simulink model "QuadRotorController_SIL"  (R2014b)
settings: Solver=FixedStepDiscrete  StartTime=0.0  StopTime=15  FixedStep=0.01  RelTol=1e-3
libraries: simulink x6
settings Model: Creator=ppreethi  LastModifiedBy=syoon
settings DataIOCC: SaveOutput=off  SaveTime=off
settings OptimizationCC: OptimizeModelRefInitCode=on  LifeSpan=Inf
settings DebuggingCC: UnderspecifiedInitializationDetection=Classic  MergeDetectMultiDrivingBlocksExec=none  StateNameClashWarn=warning
settings RTWCC: SystemTargetFile=ert.tlc  TemplateMakefile=ert_default_tmf  Description=Embedded Coder  GenerateReport=on  ProcessScript=ert_make_rtw_hook  IncludeHyperlinkInReport=on  LaunchReport=on  PortableWordSizes=on  CreateSILPILBlock=SIL  GenerateTraceInfo=on  GenerateTraceReport=on  GenerateTraceReportSl=on  GenerateTraceReportSf=on  GenerateTraceReportEml=on  GenerateCodeMetricsReport=on
settings CodeAppCC: IgnoreCustomStorageClasses=off
settings ERTTargetCC: GenerateSampleERTMain=on  SupportAbsoluteTime=off  SupportNonFinite=off  SupportComplex=off  ERTCustomFileTemplate=example_file_process.tlc
settings SimscapeCC: SelectedTab=SimMechanics2G

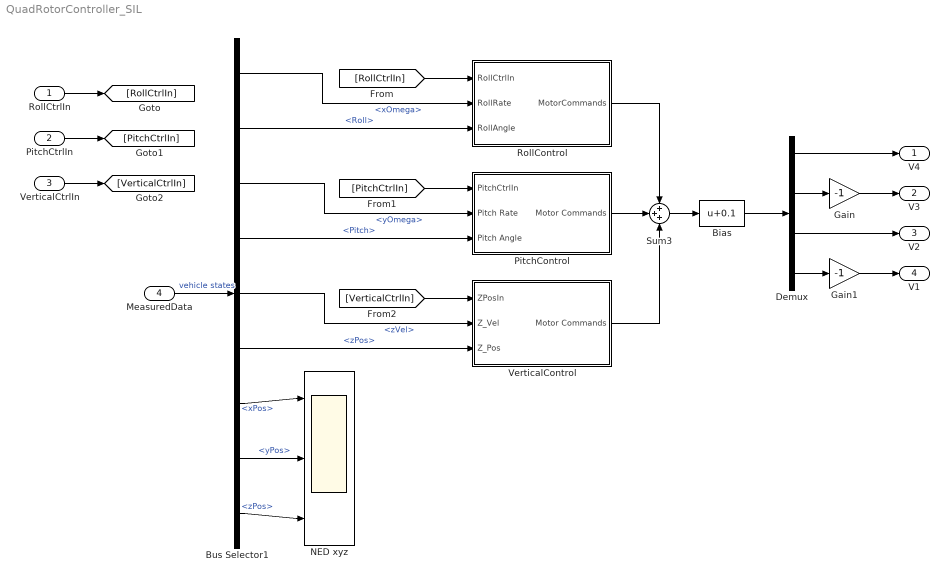
== system QuadRotorController_SIL ==
  RollCtrlIn : Inport  OutDataTypeStr=double  PortDimensions=1  SampleTime=[0.01,0]
  PitchCtrlIn : Inport  Port=2  OutDataTypeStr=double  PortDimensions=1  SampleTime=[0.01,0]
  VerticalCtrlIn : Inport  Port=3  OutDataTypeStr=double  PortDimensions=1  SampleTime=[0.01,0]
  MeasuredData : Inport  Port=4  OutDataTypeStr=Bus: VehicleStates  PortDimensions=1  SampleTime=0.01  BusOutputAsStruct=on
  Bias : Bias  Bias=0.1
  Bus Selector1 : BusSelector  OutputSignals=BodyState.AngularRate.xOmega,BodyState.Attitude.Roll,BodyState.AngularRate.yOmega,BodyState.Attitude.Pitch,BodyState.Velocity.zVel,BodyState.Position.zPos,NEDState.Position.xPos,NEDState.Position.yPos,NEDState.Position.zPos
  Demux : Demux
  Gain : Gain  Gain=-1
  Gain1 : Gain  Gain=-1
  NED xyz : Scope  NumInputPorts=3
      settings: YMin=-0.06~0.01~-1.15  YMax=0.08~0.035~-1.1  SaveName=ScopeData10
  PitchControl : Subsystem
  RollControl : Subsystem
  Sum3 : Sum  Inputs=+++
  VerticalControl : Subsystem
  V4 : Outport  OutDataTypeStr=double  PortDimensions=1  SampleTime=[0.01,0]
  V3 : Outport  Port=2  OutDataTypeStr=double  PortDimensions=1  SampleTime=[0.01,0]
  V2 : Outport  Port=3  OutDataTypeStr=double  PortDimensions=1  SampleTime=[0.01,0]
  V1 : Outport  Port=4  OutDataTypeStr=double  PortDimensions=1  SampleTime=[0.01,0]
  wires:
  Demux/3 -> V2/1
  Gain/1 -> V3/1
  Demux/2 -> Gain/1
  MeasuredData/1 -> Bus Selector1/1  "vehicle states"
  Demux/1 -> V4/1
  Gain1/1 -> V1/1
  Demux/4 -> Gain1/1
  Bus Selector1/1 -> RollControl/2(RollRate)  "<xOmega>"
  Bus Selector1/2 -> RollControl/3(RollAngle)  "<Roll>"
  Bus Selector1/3 -> PitchControl/2(Pitch Rate)  "<yOmega>"
  Bus Selector1/4 -> PitchControl/3(Pitch Angle)  "<Pitch>"
  Bus Selector1/5 -> VerticalControl/2(Z_Vel)  "<zVel>"
  Bus Selector1/6 -> VerticalControl/3(Z_Pos)  "<zPos>"
  VerticalControl/1(Motor Commands) -> Sum3/3
  Bus Selector1/8 -> NED xyz/2  "<yPos>"
  Bus Selector1/9 -> NED xyz/3  "<zPos>"
  Bus Selector1/7 -> NED xyz/1  "<xPos>"
  PitchControl/1(Motor Commands) -> Sum3/2
  RollControl/1(MotorCommands) -> Sum3/1
  Sum3/1 -> Bias/1
  Bias/1 -> Demux/1
  [VerticalCtrlIn] -> VerticalControl/1(ZPosIn)
  [RollCtrlIn] -> RollControl/1(RollCtrlIn)
  RollCtrlIn/1 -> [RollCtrlIn]
  PitchCtrlIn/1 -> [PitchCtrlIn]
  VerticalCtrlIn/1 -> [VerticalCtrlIn]
  [PitchCtrlIn] -> PitchControl/1(PitchCtrlIn)

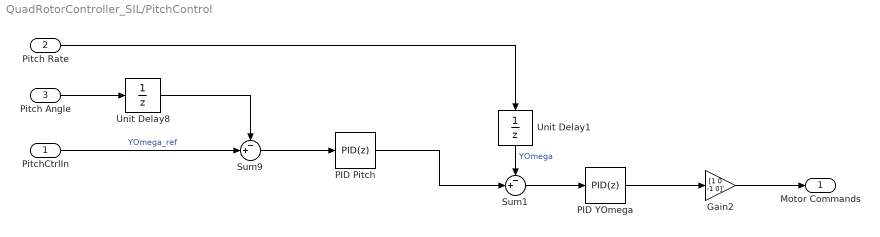
== system QuadRotorController_SIL/PitchControl ==
  PitchCtrlIn : Inport
  Pitch Rate : Inport  Port=2
  Pitch Angle : Inport  Port=3
  " PID Pitch" : simulink/Continuous/PID Controller  Controller=PID  TimeDomain=Discrete-time  SampleTime=0.01  IntegratorMethod=Forward Euler  FilterMethod=Forward Euler  Form=Parallel  P=14.2867013608458  I=2.05995750811476  D=0.849494683603069  N=180.961333470231  InitialConditionSource=internal  InitialConditionForIntegrator=0  InitialConditionForFilter=0  ExternalReset=none  LimitOutput=on  UpperSaturationLimit=10*pi/180  LowerSaturationLimit=-10*pi/180  LinearizeAsGain=on  AntiWindupMode=clamping  Kb=1  TrackingMode=off  Kt=1  PParamMin=[]  PParamMax=[]  IParamMin=[]  IParamMax=[]  DParamMin=[]  DParamMax=[]  NParamMin=[]  NParamMax=[]  KbParamMin=[]  KbParamMax=[]  KtParamMin=[]  KtParamMax=[]  POutMin=[]  POutMax=[]  IOutMin=[]  IOutMax=[]  DOutMin=[]  DOutMax=[]  NOutMin=[]  NOutMax=[]  KbOutMin=[]  KbOutMax=[]  KtOutMin=[]  KtOutMax=[]  IntegratorOutMin=[]  IntegratorOutMax=[]  FilterOutMin=[]  FilterOutMax=[]  SumOutMin=[]  SumOutMax=[]  SumI1OutMin=[]  SumI1OutMax=[]  SumI2OutMin=[]  SumI2OutMax=[]  SumI3OutMin=[]  SumI3OutMax=[]  SumDOutMin=[]  SumDOutMax=[]  SaturationOutMin=[]  SaturationOutMax=[]  IntegratorContinuousStateAttributes=''  IntegratorStateMustResolveToSignalObject=off  IntegratorRTWStateStorageClass=Auto  FilterContinuousStateAttributes=''  FilterStateMustResolveToSignalObject=off  FilterRTWStateStorageClass=Auto  DifferentiatorICPrevScaledInput=0  DifferentiatorOutMin=[]  DifferentiatorOutMax=[]  UseFilter=on
  Gain2 : Gain  Gain=[1 0 -1 0]'
  PID YOmega : simulink/Continuous/PID Controller  Controller=PID  TimeDomain=Discrete-time  SampleTime=0.01  IntegratorMethod=Forward Euler  FilterMethod=Forward Euler  Form=Parallel  P=-0.164246341346142  I=-0.0185275176619116  D=-0.032581970187069  N=81.8253210225443  InitialConditionSource=internal  InitialConditionForIntegrator=0  InitialConditionForFilter=0  ExternalReset=none  LimitOutput=on  UpperSaturationLimit=20*(pi/180)  LowerSaturationLimit=-20*(pi/180)  LinearizeAsGain=on  AntiWindupMode=clamping  Kb=1  TrackingMode=off  Kt=1  PParamMin=[]  PParamMax=[]  IParamMin=[]  IParamMax=[]  DParamMin=[]  DParamMax=[]  NParamMin=[]  NParamMax=[]  KbParamMin=[]  KbParamMax=[]  KtParamMin=[]  KtParamMax=[]  POutMin=[]  POutMax=[]  IOutMin=[]  IOutMax=[]  DOutMin=[]  DOutMax=[]  NOutMin=[]  NOutMax=[]  KbOutMin=[]  KbOutMax=[]  KtOutMin=[]  KtOutMax=[]  IntegratorOutMin=[]  IntegratorOutMax=[]  FilterOutMin=[]  FilterOutMax=[]  SumOutMin=[]  SumOutMax=[]  SumI1OutMin=[]  SumI1OutMax=[]  SumI2OutMin=[]  SumI2OutMax=[]  SumI3OutMin=[]  SumI3OutMax=[]  SumDOutMin=[]  SumDOutMax=[]  SaturationOutMin=[]  SaturationOutMax=[]  IntegratorContinuousStateAttributes=''  IntegratorStateMustResolveToSignalObject=off  IntegratorRTWStateStorageClass=Auto  FilterContinuousStateAttributes=''  FilterStateMustResolveToSignalObject=off  FilterRTWStateStorageClass=Auto  DifferentiatorICPrevScaledInput=0  DifferentiatorOutMin=[]  DifferentiatorOutMax=[]  UseFilter=on
  Sum1 : Sum  Inputs=-+|
  Sum9 : Sum  Inputs=-+|
  Unit Delay1 : UnitDelay  SampleTime=0.01
  Unit Delay8 : UnitDelay  SampleTime=0.01
  Motor Commands : Outport
  wires:
  Sum1/1 -> PID YOmega/1
  Pitch Rate/1 -> Unit Delay1/1
  Unit Delay1/1 -> Sum1/1  "YOmega"
  Pitch Angle/1 -> Unit Delay8/1
  Unit Delay8/1 -> Sum9/1
  PitchCtrlIn/1 -> Sum9/2  "YOmega_ref"
  Sum9/1 -> " PID Pitch"/1
  " PID Pitch"/1 -> Sum1/2
  PID YOmega/1 -> Gain2/1
  Gain2/1 -> Motor Commands/1

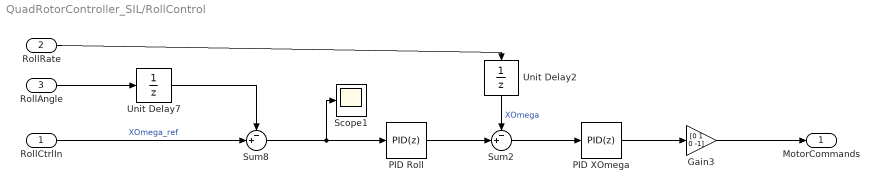
== system QuadRotorController_SIL/RollControl ==
  RollCtrlIn : Inport
  RollRate : Inport  Port=2
  RollAngle : Inport  Port=3
  " PID Roll" : simulink/Continuous/PID Controller  Controller=PID  TimeDomain=Discrete-time  SampleTime=0.01  IntegratorMethod=Forward Euler  FilterMethod=Forward Euler  Form=Parallel  P=11.7648822632631  I=1.23976611873708  D=0.415028302530751  N=77.6264609638492  InitialConditionSource=internal  InitialConditionForIntegrator=0  InitialConditionForFilter=0  ExternalReset=none  LimitOutput=on  UpperSaturationLimit=10*pi/180  LowerSaturationLimit=-10*pi/180  LinearizeAsGain=on  AntiWindupMode=clamping  Kb=1  TrackingMode=off  Kt=1  PParamMin=[]  PParamMax=[]  IParamMin=[]  IParamMax=[]  DParamMin=[]  DParamMax=[]  NParamMin=[]  NParamMax=[]  KbParamMin=[]  KbParamMax=[]  KtParamMin=[]  KtParamMax=[]  POutMin=[]  POutMax=[]  IOutMin=[]  IOutMax=[]  DOutMin=[]  DOutMax=[]  NOutMin=[]  NOutMax=[]  KbOutMin=[]  KbOutMax=[]  KtOutMin=[]  KtOutMax=[]  IntegratorOutMin=[]  IntegratorOutMax=[]  FilterOutMin=[]  FilterOutMax=[]  SumOutMin=[]  SumOutMax=[]  SumI1OutMin=[]  SumI1OutMax=[]  SumI2OutMin=[]  SumI2OutMax=[]  SumI3OutMin=[]  SumI3OutMax=[]  SumDOutMin=[]  SumDOutMax=[]  SaturationOutMin=[]  SaturationOutMax=[]  IntegratorContinuousStateAttributes=''  IntegratorStateMustResolveToSignalObject=off  IntegratorRTWStateStorageClass=Auto  FilterContinuousStateAttributes=''  FilterStateMustResolveToSignalObject=off  FilterRTWStateStorageClass=Auto  DifferentiatorICPrevScaledInput=0  DifferentiatorOutMin=[]  DifferentiatorOutMax=[]  UseFilter=on
  " PID XOmega" : simulink/Continuous/PID Controller  Controller=PID  TimeDomain=Discrete-time  SampleTime=0.01  IntegratorMethod=Forward Euler  FilterMethod=Forward Euler  Form=Parallel  P=-0.159149757061445  I=-0.0204269947322092  D=-0.0384500404495734  N=88.6017486491099  InitialConditionSource=internal  InitialConditionForIntegrator=0  InitialConditionForFilter=0  ExternalReset=none  LimitOutput=on  UpperSaturationLimit=20*(pi/180)  LowerSaturationLimit=-20*(pi/180)  LinearizeAsGain=on  AntiWindupMode=clamping  Kb=1  TrackingMode=off  Kt=1  PParamMin=[]  PParamMax=[]  IParamMin=[]  IParamMax=[]  DParamMin=[]  DParamMax=[]  NParamMin=[]  NParamMax=[]  KbParamMin=[]  KbParamMax=[]  KtParamMin=[]  KtParamMax=[]  POutMin=[]  POutMax=[]  IOutMin=[]  IOutMax=[]  DOutMin=[]  DOutMax=[]  NOutMin=[]  NOutMax=[]  KbOutMin=[]  KbOutMax=[]  KtOutMin=[]  KtOutMax=[]  IntegratorOutMin=[]  IntegratorOutMax=[]  FilterOutMin=[]  FilterOutMax=[]  SumOutMin=[]  SumOutMax=[]  SumI1OutMin=[]  SumI1OutMax=[]  SumI2OutMin=[]  SumI2OutMax=[]  SumI3OutMin=[]  SumI3OutMax=[]  SumDOutMin=[]  SumDOutMax=[]  SaturationOutMin=[]  SaturationOutMax=[]  IntegratorContinuousStateAttributes=''  IntegratorStateMustResolveToSignalObject=off  IntegratorRTWStateStorageClass=Auto  FilterContinuousStateAttributes=''  FilterStateMustResolveToSignalObject=off  FilterRTWStateStorageClass=Auto  DifferentiatorICPrevScaledInput=0  DifferentiatorOutMin=[]  DifferentiatorOutMax=[]  UseFilter=on
  Gain3 : Gain  Gain=[0 1 0 -1]
  Scope1 : Scope
      settings: YMin=-3.5  YMax=3.5  SaveName=ScopeData5
  Sum2 : Sum  Inputs=-+|
  Sum8 : Sum  Inputs=-+|
  Unit Delay2 : UnitDelay  SampleTime=0.01
  Unit Delay7 : UnitDelay  SampleTime=0.01
  MotorCommands : Outport
  wires:
  Gain3/1 -> MotorCommands/1
  Unit Delay2/1 -> Sum2/1  "XOmega"
  RollRate/1 -> Unit Delay2/1
  Sum2/1 -> " PID XOmega"/1
  " PID XOmega"/1 -> Gain3/1
  " PID Roll"/1 -> Sum2/2
  Unit Delay7/1 -> Sum8/1
  Sum8/1 -> " PID Roll"/1, Scope1/1
  RollAngle/1 -> Unit Delay7/1
  RollCtrlIn/1 -> Sum8/2  "XOmega_ref"

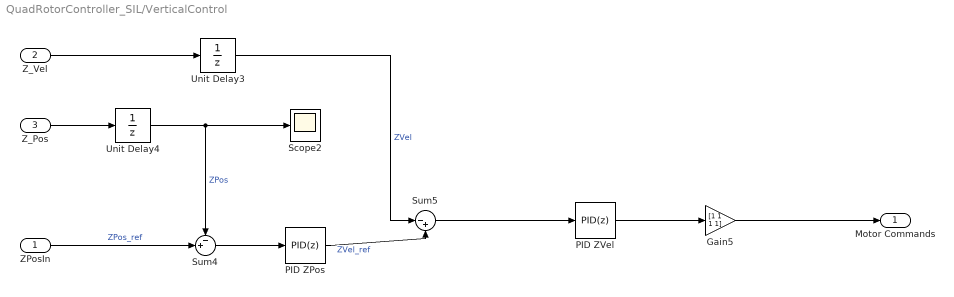
== system QuadRotorController_SIL/VerticalControl ==
  ZPosIn : Inport
  Z_Vel : Inport  Port=2
  Z_Pos : Inport  Port=3
  Gain5 : Gain  Gain=[1 1 1 1]
  PID ZPos : simulink/Continuous/PID Controller  Controller=PID  TimeDomain=Discrete-time  SampleTime=0.01  IntegratorMethod=Forward Euler  FilterMethod=Forward Euler  Form=Parallel  P=15.2064009134149  I=2.28704553088529  D=1.26307161184834  N=181.743667624326  InitialConditionSource=internal  InitialConditionForIntegrator=0  InitialConditionForFilter=0  ExternalReset=none  LimitOutput=on  UpperSaturationLimit=2  LowerSaturationLimit=-0  LinearizeAsGain=on  AntiWindupMode=none  Kb=1  TrackingMode=off  Kt=1  PParamMin=[]  PParamMax=[]  IParamMin=[]  IParamMax=[]  DParamMin=[]  DParamMax=[]  NParamMin=[]  NParamMax=[]  KbParamMin=[]  KbParamMax=[]  KtParamMin=[]  KtParamMax=[]  POutMin=[]  POutMax=[]  IOutMin=[]  IOutMax=[]  DOutMin=[]  DOutMax=[]  NOutMin=[]  NOutMax=[]  KbOutMin=[]  KbOutMax=[]  KtOutMin=[]  KtOutMax=[]  IntegratorOutMin=[]  IntegratorOutMax=[]  FilterOutMin=[]  FilterOutMax=[]  SumOutMin=[]  SumOutMax=[]  SumI1OutMin=[]  SumI1OutMax=[]  SumI2OutMin=[]  SumI2OutMax=[]  SumI3OutMin=[]  SumI3OutMax=[]  SumDOutMin=[]  SumDOutMax=[]  SaturationOutMin=[]  SaturationOutMax=[]  IntegratorContinuousStateAttributes=''  IntegratorStateMustResolveToSignalObject=off  IntegratorRTWStateStorageClass=Auto  FilterContinuousStateAttributes=''  FilterStateMustResolveToSignalObject=off  FilterRTWStateStorageClass=Auto  DifferentiatorICPrevScaledInput=0  DifferentiatorOutMin=[]  DifferentiatorOutMax=[]  UseFilter=on
  PID ZVel : simulink/Continuous/PID Controller  Controller=PID  TimeDomain=Discrete-time  SampleTime=0.01  IntegratorMethod=Forward Euler  FilterMethod=Forward Euler  Form=Parallel  P=2.57661196228208  I=1.40117055525367  D=0.595498757922882  N=68.7884382089654  InitialConditionSource=internal  InitialConditionForIntegrator=0  InitialConditionForFilter=0  ExternalReset=none  LimitOutput=off  UpperSaturationLimit=inf  LowerSaturationLimit=-inf  LinearizeAsGain=on  AntiWindupMode=none  Kb=1  TrackingMode=off  Kt=1  PParamMin=[]  PParamMax=[]  IParamMin=[]  IParamMax=[]  DParamMin=[]  DParamMax=[]  NParamMin=[]  NParamMax=[]  KbParamMin=[]  KbParamMax=[]  KtParamMin=[]  KtParamMax=[]  POutMin=[]  POutMax=[]  IOutMin=[]  IOutMax=[]  DOutMin=[]  DOutMax=[]  NOutMin=[]  NOutMax=[]  KbOutMin=[]  KbOutMax=[]  KtOutMin=[]  KtOutMax=[]  IntegratorOutMin=[]  IntegratorOutMax=[]  FilterOutMin=[]  FilterOutMax=[]  SumOutMin=[]  SumOutMax=[]  SumI1OutMin=[]  SumI1OutMax=[]  SumI2OutMin=[]  SumI2OutMax=[]  SumI3OutMin=[]  SumI3OutMax=[]  SumDOutMin=[]  SumDOutMax=[]  SaturationOutMin=[]  SaturationOutMax=[]  IntegratorContinuousStateAttributes=''  IntegratorStateMustResolveToSignalObject=off  IntegratorRTWStateStorageClass=Auto  FilterContinuousStateAttributes=''  FilterStateMustResolveToSignalObject=off  FilterRTWStateStorageClass=Auto  DifferentiatorICPrevScaledInput=0  DifferentiatorOutMin=[]  DifferentiatorOutMax=[]  UseFilter=on
  Scope2 : Scope
      settings: YMin=-1.8  YMax=0.6  SaveName=ScopeData6
  Sum4 : Sum  Inputs=-+|
  Sum5 : Sum  Inputs=|-+
  Unit Delay3 : UnitDelay  SampleTime=0.01
  Unit Delay4 : UnitDelay  SampleTime=0.01
  Motor Commands : Outport
  wires:
  Sum5/1 -> PID ZVel/1
  PID ZPos/1 -> Sum5/2  "ZVel_ref"
  Unit Delay3/1 -> Sum5/1  "ZVel"
  Gain5/1 -> Motor Commands/1
  PID ZVel/1 -> Gain5/1
  Unit Delay4/1 -> Scope2/1, Sum4/1  "ZPos"
  Z_Pos/1 -> Unit Delay4/1
  ZPosIn/1 -> Sum4/2  "ZPos_ref"
  Z_Vel/1 -> Unit Delay3/1
  Sum4/1 -> PID ZPos/1
